simulink library "VIS_LIB"  (Simulink 8.6)
settings: Solver=ode45  StartTime=0.0  StopTime=10.0  RelTol=1e-3
undefined symbols (not defined in the file): AC, SIXOSEM_F_WD_AC_MASTER
libraries: cdsFilt x376, cdsEpicsOut x253, cdsEpicsIn x179, cdsTP x123, VIS_LIB x95, cdsMuxMatrix x91, cdsEpicsStringIn x75, cdsFiltCtrl x72, cdsFunctionCall x70, cdsRms x59, KAGRA_UTIL x25, STATE_BIO_MASTER x5
(part 30 of 38)

== system VIS_LIB/MODAL/inputproc_forQUA/OL_PROC ==
  MNSEG1 : Inport
  MNSEG2 : Inport  Port=2
  MNSEG3 : Inport  Port=3
  MNSEG4 : Inport  Port=4
  TILT_SEG1 : Inport  Port=5
  TILT_SEG2 : Inport  Port=6
  TILT_SEG3 : Inport  Port=7
  TILT_SEG4 : Inport  Port=8
  LEN_SEG1 : Inport  Port=9
  LEN_SEG2 : Inport  Port=10
  LEN_SEG3 : Inport  Port=11
  LEN_SEG4 : Inport  Port=12
  MN_TILT : VIS_LIB/UTILs/OL
  TM_LEN : VIS_LIB/UTILs/OL
  TM_TILT : VIS_LIB/UTILs/OL
  MNV : Outport
  MNH : Outport  Port=2
  TMV1 : Outport  Port=3
  TMV2 : Outport  Port=4
  TMH1 : Outport  Port=5
  TMH2 : Outport  Port=6
  wires:
  MNSEG2/1 -> MN_TILT/2
  MNSEG1/1 -> MN_TILT/1
  MNSEG4/1 -> MN_TILT/4
  MN_TILT/1 -> MNV/1
  MN_TILT/2 -> MNH/1
  MNSEG3/1 -> MN_TILT/3
  TILT_SEG1/1 -> TM_TILT/1
  TILT_SEG2/1 -> TM_TILT/2
  TILT_SEG4/1 -> TM_TILT/4
  TILT_SEG3/1 -> TM_TILT/3
  LEN_SEG1/1 -> TM_LEN/1
  LEN_SEG2/1 -> TM_LEN/2
  LEN_SEG3/1 -> TM_LEN/3
  LEN_SEG4/1 -> TM_LEN/4
  TM_TILT/1 -> TMV1/1
  TM_TILT/2 -> TMH1/1
  TM_LEN/1 -> TMV2/1
  TM_LEN/2 -> TMH2/1

== system VIS_LIB/MODAL/inputproc_forQUA/SEN2EUL ==
  In1 : Inport
  In2 : Inport  Port=2
  In3 : Inport  Port=3
  In4 : Inport  Port=4
  In5 : Inport  Port=5
  In6 : Inport  Port=6
  In7 : Inport  Port=7
  In8 : Inport  Port=8
  In9 : Inport  Port=9
  In10 : Inport  Port=10
  In11 : Inport  Port=11
  In12 : Inport  Port=12
  In13 : Inport  Port=13
  In14 : Inport  Port=14
  In15 : Inport  Port=15
  In20 : Inport  Port=16
  In21 : Inport  Port=17
  In22 : Inport  Port=18
  In27 : Inport  Port=19
  In28 : Inport  Port=20
  In29 : Inport  Port=21
  In30 : Inport  Port=22
  In31 : Inport  Port=23
  In32 : Inport  Port=24
  In33 : Inport  Port=25
  In34 : Inport  Port=26
  In35 : Inport  Port=27
  In36 : Inport  Port=28
  In37 : Inport  Port=29
  In38 : Inport  Port=30
  In16 : Inport  Port=31
  In17 : Inport  Port=32
  In18 : Inport  Port=33
  In19 : Inport  Port=34
  In23 : Inport  Port=35
  In24 : Inport  Port=36
  BF : cdsMuxMatrix/Subsystem  Tag=cdsMuxMatrix  Description=Any size matrix. Inputs and outputs must be connected using Mux and Demux parts.
      settings: AttributesFormatString=%<Tag>
  Demux{1..6} (6 alike) : Demux  Outputs=6
  IM : cdsMuxMatrix/Subsystem  Tag=cdsMuxMatrix  Description=Any size matrix. Inputs and outputs must be connected using Mux and Demux parts.
      settings: AttributesFormatString=%<Tag>
  IP : cdsMuxMatrix/Subsystem  Tag=cdsMuxMatrix  Description=Any size matrix. Inputs and outputs must be connected using Mux and Demux parts.
      settings: AttributesFormatString=%<Tag>
  MN : cdsMuxMatrix/Subsystem  Tag=cdsMuxMatrix  Description=Any size matrix. Inputs and outputs must be connected using Mux and Demux parts.
      settings: AttributesFormatString=%<Tag>
  MNOL : cdsMuxMatrix/Subsystem  Tag=cdsMuxMatrix  Description=Any size matrix. Inputs and outputs must be connected using Mux and Demux parts.
      settings: AttributesFormatString=%<Tag>
  Mux{1..6} (6 alike) : Mux  Inputs=6
  TM : cdsMuxMatrix/Subsystem  Tag=cdsMuxMatrix  Description=Any size matrix. Inputs and outputs must be connected using Mux and Demux parts.
      settings: AttributesFormatString=%<Tag>
  IPLo : Outport
  IPTo : Outport  Port=2
  IPVo : Outport  Port=3
  IPRo : Outport  Port=4
  IPPo : Outport  Port=5
  IPYo : Outport  Port=6
  BFLo : Outport  Port=7
  BFTo : Outport  Port=8
  BFVo : Outport  Port=9
  BFRo : Outport  Port=10
  BFPo : Outport  Port=11
  BFYo : Outport  Port=12
  MNLo : Outport  Port=13
  MNTo : Outport  Port=14
  MNVo : Outport  Port=15
  MNRo : Outport  Port=16
  MNPo : Outport  Port=17
  MNYo : Outport  Port=18
  IMLo : Outport  Port=19
  IMTo : Outport  Port=20
  IMVo : Outport  Port=21
  IMRo : Outport  Port=22
  IMPo : Outport  Port=23
  IMYo : Outport  Port=24
  TMLo : Outport  Port=25
  TMTo : Outport  Port=26
  TMVo : Outport  Port=27
  TMRo : Outport  Port=28
  TMPop : Outport  Port=29
  TMYo : Outport  Port=30
  TMLo1 : Outport  Port=31
  TMTo1 : Outport  Port=32
  TMVo1 : Outport  Port=33
  TMRo1 : Outport  Port=34
  TMPop1 : Outport  Port=35
  TMYo1 : Outport  Port=36
  wires:
  In6/1 -> Mux2/6
  Mux2/1 -> IP/1
  In3/1 -> Mux2/3
  In1/1 -> Mux2/1
  IP/1 -> Demux3/1
  In5/1 -> Mux2/5
  In2/1 -> Mux2/2
  In4/1 -> Mux2/4
  In12/1 -> Mux1/6
  Mux1/1 -> BF/1
  In9/1 -> Mux1/3
  In7/1 -> Mux1/1
  BF/1 -> Demux1/1
  In11/1 -> Mux1/5
  In8/1 -> Mux1/2
  In10/1 -> Mux1/4
  Mux3/1 -> MN/1
  In15/1 -> Mux3/3
  In13/1 -> Mux3/1
  MN/1 -> Demux2/1
  In14/1 -> Mux3/2
  Mux4/1 -> IM/1
  IM/1 -> Demux4/1
  In21/1 -> Mux3/5
  In20/1 -> Mux3/4
  In22/1 -> Mux3/6
  In30/1 -> Mux4/4
  In27/1 -> Mux4/1
  In29/1 -> Mux4/3
  In28/1 -> Mux4/2
  In32/1 -> Mux4/6
  In31/1 -> Mux4/5
  In38/1 -> Mux5/6
  Mux5/1 -> TM/1
  In35/1 -> Mux5/3
  In33/1 -> Mux5/1
  TM/1 -> Demux5/1
  In37/1 -> Mux5/5
  In34/1 -> Mux5/2
  In36/1 -> Mux5/4
  Demux3/6 -> IPYo/1
  Demux1/1 -> BFLo/1
  Demux1/2 -> BFTo/1
  Demux1/3 -> BFVo/1
  Demux1/4 -> BFRo/1
  Demux1/5 -> BFPo/1
  Demux1/6 -> BFYo/1
  Demux2/1 -> MNLo/1
  Demux2/2 -> MNTo/1
  Demux2/3 -> MNVo/1
  Demux2/4 -> MNRo/1
  Demux2/5 -> MNPo/1
  Demux2/6 -> MNYo/1
  Demux4/1 -> IMLo/1
  Demux4/2 -> IMTo/1
  Demux4/3 -> IMVo/1
  Demux4/4 -> IMRo/1
  Demux4/5 -> IMPo/1
  Demux4/6 -> IMYo/1
  Demux5/1 -> TMLo/1
  Demux3/1 -> IPLo/1
  Demux3/2 -> IPTo/1
  Demux3/3 -> IPVo/1
  Demux3/4 -> IPRo/1
  Demux3/5 -> IPPo/1
  Demux5/2 -> TMTo/1
  Demux5/3 -> TMVo/1
  Demux5/4 -> TMRo/1
  Demux5/5 -> TMPop/1
  Demux5/6 -> TMYo/1
  In24/1 -> Mux6/6
  Mux6/1 -> MNOL/1
  In18/1 -> Mux6/3
  MNOL/1 -> Demux6/1
  In23/1 -> Mux6/5
  In17/1 -> Mux6/2
  In19/1 -> Mux6/4
  Demux6/2 -> TMTo1/1
  Demux6/3 -> TMVo1/1
  Demux6/4 -> TMRo1/1
  Demux6/5 -> TMPop1/1
  Demux6/6 -> TMYo1/1
  Demux6/1 -> TMLo1/1
  In16/1 -> Mux6/1

== system VIS_LIB/MODAL/inputproc_forQUA/SENSIN ==
  IPLVDT_H1 : Inport
  IPLVDT_H2 : Inport  Port=2
  IPLVDT_H3 : Inport  Port=3
  BFLVDT_V1 : Inport  Port=4
  BFLVDT_V2 : Inport  Port=5
  BFLVDT_V3 : Inport  Port=6
  BFLVDT_H1 : Inport  Port=7
  BFLVDT_H2 : Inport  Port=8
  BFLVDT_H3 : Inport  Port=9
  MCPS_V1 : Inport  Port=10
  MCPS_V2 : Inport  Port=11
  MCPS_V3 : Inport  Port=12
  MCPS_H1 : Inport  Port=13
  MCPS_H2 : Inport  Port=14
  MNPS_H3 : Inport  Port=15
  IMPS_V1 : Inport  Port=16
  IMPS_V2 : Inport  Port=17
  IMPS_V3 : Inport  Port=18
  IMPS_H1 : Inport  Port=19
  IMPS_H2 : Inport  Port=20
  IMPS_H3 : Inport  Port=21
  MNOL_V : Inport  Port=22
  MNOL_H4 : Inport  Port=23
  TMOLV1 : Inport  Port=24
  TMOLV2 : Inport  Port=25
  TMOLH1 : Inport  Port=26
  TMOLH2 : Inport  Port=27
  BF : VIS_LIB/UTILs/6COILs_DQ
  Ground{1..7,9..10} (9 alike) : Ground
  IM : VIS_LIB/UTILs/6COILs_DQ
  IP : VIS_LIB/UTILs/6COILs_DQ
  MN : VIS_LIB/UTILs/6COILs_DQ
  MNOL : VIS_LIB/UTILs/6COILs_DQ
  TM : VIS_LIB/UTILs/6COILs_DQ
  IPV1 : Outport
  IPV2 : Outport  Port=2
  IPV3 : Outport  Port=3
  IPH1 : Outport  Port=4
  IPH2 : Outport  Port=5
  IPH3 : Outport  Port=6
  BFV1 : Outport  Port=7
  BFV2 : Outport  Port=8
  BFV3 : Outport  Port=9
  BFH1 : Outport  Port=10
  BFH2 : Outport  Port=11
  BFH3 : Outport  Port=12
  MNV1 : Outport  Port=13
  MNV2 : Outport  Port=14
  MNV3 : Outport  Port=15
  MNH1 : Outport  Port=16
  MNH2 : Outport  Port=17
  MNH3 : Outport  Port=18
  IMV1 : Outport  Port=19
  IMV2 : Outport  Port=20
  IMV3 : Outport  Port=21
  IMH1 : Outport  Port=22
  IMH2 : Outport  Port=23
  IMH3 : Outport  Port=24
  IMV4 : Outport  Port=25
  IMV5 : Outport  Port=26
  IMV6 : Outport  Port=27
  IMH4 : Outport  Port=28
  IMH5 : Outport  Port=29
  IMH6 : Outport  Port=30
  MNOLV1 : Outport  Port=31
  MNOLV2 : Outport  Port=32
  MNOLV3 : Outport  Port=33
  MNOLH1 : Outport  Port=34
  MNOLH2 : Outport  Port=35
  MNOLH3 : Outport  Port=36
  wires:
  IPLVDT_H1/1 -> IP/4
  IPLVDT_H2/1 -> IP/5
  IPLVDT_H3/1 -> IP/6
  BFLVDT_V1/1 -> BF/1
  BFLVDT_V2/1 -> BF/2
  BFLVDT_V3/1 -> BF/3
  BFLVDT_H1/1 -> BF/4
  BFLVDT_H2/1 -> BF/5
  BFLVDT_H3/1 -> BF/6
  MCPS_V1/1 -> MN/1
  MCPS_V2/1 -> MN/2
  MCPS_V3/1 -> MN/3
  MCPS_H1/1 -> MN/4
  MCPS_H2/1 -> MN/5
  MNPS_H3/1 -> MN/6
  IMPS_V1/1 -> IM/1
  IMPS_V2/1 -> IM/2
  IMPS_V3/1 -> IM/3
  IMPS_H1/1 -> IM/4
  IMPS_H2/1 -> IM/5
  IMPS_H3/1 -> IM/6
  Ground2/1 -> IP/1
  Ground1/1 -> IP/2
  Ground3/1 -> IP/3
  IP/5 -> IPH2/1
  IP/4 -> IPH1/1
  IP/6 -> IPH3/1
  BF/1 -> BFV1/1
  BF/3 -> BFV3/1
  BF/5 -> BFH2/1
  BF/6 -> BFH3/1
  BF/2 -> BFV2/1
  BF/4 -> BFH1/1
  IM/6 -> IMH3/1
  IM/5 -> IMH2/1
  IM/4 -> IMH1/1
  IM/3 -> IMV3/1
  IM/2 -> IMV2/1
  IM/1 -> IMV1/1
  MN/6 -> MNH3/1
  MN/5 -> MNH2/1
  MN/4 -> MNH1/1
  MN/3 -> MNV3/1
  MN/2 -> MNV2/1
  MN/1 -> MNV1/1
  IP/1 -> IPV1/1
  IP/2 -> IPV2/1
  IP/3 -> IPV3/1
  MNOL_V/1 -> MNOL/1
  MNOL_H4/1 -> MNOL/4
  TMOLV2/1 -> TM/2
  TMOLH1/1 -> TM/4
  TMOLH2/1 -> TM/5
  TM/6 -> IMH6/1
  TM/5 -> IMH5/1
  TM/4 -> IMH4/1
  TM/3 -> IMV6/1
  TM/2 -> IMV5/1
  TMOLV1/1 -> TM/1
  Ground9/1 -> TM/3
  Ground10/1 -> TM/6
  TM/1 -> IMV4/1
  MNOL/6 -> MNOLH3/1
  MNOL/5 -> MNOLH2/1
  MNOL/4 -> MNOLH1/1
  MNOL/3 -> MNOLV3/1
  MNOL/2 -> MNOLV2/1
  Ground5/1 -> MNOL/3
  Ground4/1 -> MNOL/6
  MNOL/1 -> MNOLV1/1
  Ground7/1 -> MNOL/2
  Ground6/1 -> MNOL/5

== system VIS_LIB/MODAL/inputproc_forQUA/SENSIN_GAS ==
  note: #DAQ Channels
      |
      | F0_OUT 256
      | F1_OUT 256
      | F2_OUT 256
      | F3_OUT 256
      | BF_OUT 256
  iF0 : Inport
  iF1 : Inport  Port=2
  iF2 : Inport  Port=3
  iF3 : Inport  Port=4
  iBF : Inport  Port=5
  BF : cdsFilt/Subsystem  Tag=cdsFilt  Description=|
      | Purpose:                                                                                                                                                                                                                                  
      | Standard CDS IIR filter module.                                                                                                                                                                                                           
      |                                                                                                                                                                                                                                           
      | Operation:                                                                                                                                                                                                                                
      | Consists of 10 second order section IIR filters, plus a ramped gain stage. In FE code, also provides pre-defined test points and excitation channel inputs. The filter coefficients are defined in the LIGO system using the 'foton' tool.
      |                                                                                                                                                                                                                                           
      | Usage:                                                                                                                                                                                                                                    
      | Name the part with the desired filter module name.
      settings: AttributesFormatString=%<Tag>
  F0 : cdsFilt/Subsystem  Tag=cdsFilt  Description=|
      | Purpose:                                                                                                                                                                                                                                  
      | Standard CDS IIR filter module.                                                                                                                                                                                                           
      |                                                                                                                                                                                                                                           
      | Operation:                                                                                                                                                                                                                                
      | Consists of 10 second order section IIR filters, plus a ramped gain stage. In FE code, also provides pre-defined test points and excitation channel inputs. The filter coefficients are defined in the LIGO system using the 'foton' tool.
      |                                                                                                                                                                                                                                           
      | Usage:                                                                                                                                                                                                                                    
      | Name the part with the desired filter module name.
      settings: AttributesFormatString=%<Tag>
  F1 : cdsFilt/Subsystem  Tag=cdsFilt  Description=|
      | Purpose:                                                                                                                                                                                                                                  
      | Standard CDS IIR filter module.                                                                                                                                                                                                           
      |                                                                                                                                                                                                                                           
      | Operation:                                                                                                                                                                                                                                
      | Consists of 10 second order section IIR filters, plus a ramped gain stage. In FE code, also provides pre-defined test points and excitation channel inputs. The filter coefficients are defined in the LIGO system using the 'foton' tool.
      |                                                                                                                                                                                                                                           
      | Usage:                                                                                                                                                                                                                                    
      | Name the part with the desired filter module name.
      settings: AttributesFormatString=%<Tag>
  F2 : cdsFilt/Subsystem  Tag=cdsFilt  Description=|
      | Purpose:                                                                                                                                                                                                                                  
      | Standard CDS IIR filter module.                                                                                                                                                                                                           
      |                                                                                                                                                                                                                                           
      | Operation:                                                                                                                                                                                                                                
      | Consists of 10 second order section IIR filters, plus a ramped gain stage. In FE code, also provides pre-defined test points and excitation channel inputs. The filter coefficients are defined in the LIGO system using the 'foton' tool.
      |                                                                                                                                                                                                                                           
      | Usage:                                                                                                                                                                                                                                    
      | Name the part with the desired filter module name.
      settings: AttributesFormatString=%<Tag>
  F3 : cdsFilt/Subsystem  Tag=cdsFilt  Description=|
      | Purpose:                                                                                                                                                                                                                                  
      | Standard CDS IIR filter module.                                                                                                                                                                                                           
      |                                                                                                                                                                                                                                           
      | Operation:                                                                                                                                                                                                                                
      | Consists of 10 second order section IIR filters, plus a ramped gain stage. In FE code, also provides pre-defined test points and excitation channel inputs. The filter coefficients are defined in the LIGO system using the 'foton' tool.
      |                                                                                                                                                                                                                                           
      | Usage:                                                                                                                                                                                                                                    
      | Name the part with the desired filter module name.
      settings: AttributesFormatString=%<Tag>
  oF0 : Outport
  oF1 : Outport  Port=2
  oF2 : Outport  Port=3
  oF3 : Outport  Port=4
  oBF : Outport  Port=5
  wires:
  BF/1 -> oBF/1
  iBF/1 -> BF/1
  F3/1 -> oF3/1
  iF3/1 -> F3/1
  F2/1 -> oF2/1
  iF2/1 -> F2/1
  F1/1 -> oF1/1
  iF1/1 -> F1/1
  F0/1 -> oF0/1
  iF0/1 -> F0/1

== system VIS_LIB/WD2/AC/BANDLIM ==
  F0_In : Inport
  SF_In : Inport  Port=2
  BF_In : Inport  Port=3
  BF : cdsFilt/Subsystem  Tag=cdsFilt  Description=|
      | Purpose:                                                                                                                                                                                                                                  
      | Standard CDS IIR filter module.                                                                                                                                                                                                           
      |                                                                                                                                                                                                                                           
      | Operation:                                                                                                                                                                                                                                
      | Consists of 10 second order section IIR filters, plus a ramped gain stage. In FE code, also provides pre-defined test points and excitation channel inputs. The filter coefficients are defined in the LIGO system using the 'foton' tool.
      |                                                                                                                                                                                                                                           
      | Usage:                                                                                                                                                                                                                                    
      | Name the part with the desired filter module name.
      settings: AttributesFormatString=%<Tag>
  F0 : cdsFilt/Subsystem  Tag=cdsFilt  Description=|
      | Purpose:                                                                                                                                                                                                                                  
      | Standard CDS IIR filter module.                                                                                                                                                                                                           
      |                                                                                                                                                                                                                                           
      | Operation:                                                                                                                                                                                                                                
      | Consists of 10 second order section IIR filters, plus a ramped gain stage. In FE code, also provides pre-defined test points and excitation channel inputs. The filter coefficients are defined in the LIGO system using the 'foton' tool.
      |                                                                                                                                                                                                                                           
      | Usage:                                                                                                                                                                                                                                    
      | Name the part with the desired filter module name.
      settings: AttributesFormatString=%<Tag>
  SF : cdsFilt/Subsystem  Tag=cdsFilt  Description=|
      | Purpose:                                                                                                                                                                                                                                  
      | Standard CDS IIR filter module.                                                                                                                                                                                                           
      |                                                                                                                                                                                                                                           
      | Operation:                                                                                                                                                                                                                                
      | Consists of 10 second order section IIR filters, plus a ramped gain stage. In FE code, also provides pre-defined test points and excitation channel inputs. The filter coefficients are defined in the LIGO system using the 'foton' tool.
      |                                                                                                                                                                                                                                           
      | Usage:                                                                                                                                                                                                                                    
      | Name the part with the desired filter module name.
      settings: AttributesFormatString=%<Tag>
  F0_Out : Outport
  SF_Out : Outport  Port=2
  BF_Out : Outport  Port=3
  wires:
  BF/1 -> BF_Out/1
  BF_In/1 -> BF/1
  SF/1 -> SF_Out/1
  SF_In/1 -> SF/1
  F0/1 -> F0_Out/1
  F0_In/1 -> F0/1

== system VIS_LIB/WD3/OSEMAC/BANDLIM ==
  V1_In : Inport
  V2_In : Inport  Port=2
  V3_In : Inport  Port=3
  H1_In : Inport  Port=4
  H2_In : Inport  Port=5
  H3_In : Inport  Port=6
  H1 : cdsFilt/Subsystem  Tag=cdsFilt  Description=|
      | Purpose:                                                                                                                                                                                                                                  
      | Standard CDS IIR filter module.                                                                                                                                                                                                           
      |                                                                                                                                                                                                                                           
      | Operation:                                                                                                                                                                                                                                
      | Consists of 10 second order section IIR filters, plus a ramped gain stage. In FE code, also provides pre-defined test points and excitation channel inputs. The filter coefficients are defined in the LIGO system using the 'foton' tool.
      |                                                                                                                                                                                                                                           
      | Usage:                                                                                                                                                                                                                                    
      | Name the part with the desired filter module name.
      settings: AttributesFormatString=%<Tag>
  H2 : cdsFilt/Subsystem  Tag=cdsFilt  Description=|
      | Purpose:                                                                                                                                                                                                                                  
      | Standard CDS IIR filter module.                                                                                                                                                                                                           
      |                                                                                                                                                                                                                                           
      | Operation:                                                                                                                                                                                                                                
      | Consists of 10 second order section IIR filters, plus a ramped gain stage. In FE code, also provides pre-defined test points and excitation channel inputs. The filter coefficients are defined in the LIGO system using the 'foton' tool.
      |                                                                                                                                                                                                                                           
      | Usage:                                                                                                                                                                                                                                    
      | Name the part with the desired filter module name.
      settings: AttributesFormatString=%<Tag>
  H3 : cdsFilt/Subsystem  Tag=cdsFilt  Description=|
      | Purpose:                                                                                                                                                                                                                                  
      | Standard CDS IIR filter module.                                                                                                                                                                                                           
      |                                                                                                                                                                                                                                           
      | Operation:                                                                                                                                                                                                                                
      | Consists of 10 second order section IIR filters, plus a ramped gain stage. In FE code, also provides pre-defined test points and excitation channel inputs. The filter coefficients are defined in the LIGO system using the 'foton' tool.
      |                                                                                                                                                                                                                                           
      | Usage:                                                                                                                                                                                                                                    
      | Name the part with the desired filter module name.
      settings: AttributesFormatString=%<Tag>
  V1 : cdsFilt/Subsystem  Tag=cdsFilt  Description=|
      | Purpose:                                                                                                                                                                                                                                  
      | Standard CDS IIR filter module.                                                                                                                                                                                                           
      |                                                                                                                                                                                                                                           
      | Operation:                                                                                                                                                                                                                                
      | Consists of 10 second order section IIR filters, plus a ramped gain stage. In FE code, also provides pre-defined test points and excitation channel inputs. The filter coefficients are defined in the LIGO system using the 'foton' tool.
      |                                                                                                                                                                                                                                           
      | Usage:                                                                                                                                                                                                                                    
      | Name the part with the desired filter module name.
      settings: AttributesFormatString=%<Tag>
  V2 : cdsFilt/Subsystem  Tag=cdsFilt  Description=|
      | Purpose:                                                                                                                                                                                                                                  
      | Standard CDS IIR filter module.                                                                                                                                                                                                           
      |                                                                                                                                                                                                                                           
      | Operation:                                                                                                                                                                                                                                
      | Consists of 10 second order section IIR filters, plus a ramped gain stage. In FE code, also provides pre-defined test points and excitation channel inputs. The filter coefficients are defined in the LIGO system using the 'foton' tool.
      |                                                                                                                                                                                                                                           
      | Usage:                                                                                                                                                                                                                                    
      | Name the part with the desired filter module name.
      settings: AttributesFormatString=%<Tag>
  V3 : cdsFilt/Subsystem  Tag=cdsFilt  Description=|
      | Purpose:                                                                                                                                                                                                                                  
      | Standard CDS IIR filter module.                                                                                                                                                                                                           
      |                                                                                                                                                                                                                                           
      | Operation:                                                                                                                                                                                                                                
      | Consists of 10 second order section IIR filters, plus a ramped gain stage. In FE code, also provides pre-defined test points and excitation channel inputs. The filter coefficients are defined in the LIGO system using the 'foton' tool.
      |                                                                                                                                                                                                                                           
      | Usage:                                                                                                                                                                                                                                    
      | Name the part with the desired filter module name.
      settings: AttributesFormatString=%<Tag>
  V1_Out : Outport
  V2_Out : Outport  Port=2
  V3_Out : Outport  Port=3
  H1_Out : Outport  Port=4
  H2_Out : Outport  Port=5
  H3_Out : Outport  Port=6
  wires:
  V1/1 -> V1_Out/1
  V2/1 -> V2_Out/1
  V3/1 -> V3_Out/1
  V1_In/1 -> V1/1
  V2_In/1 -> V2/1
  V3_In/1 -> V3/1
  H1/1 -> H1_Out/1
  H2/1 -> H2_Out/1
  H3/1 -> H3_Out/1
  H1_In/1 -> H1/1
  H2_In/1 -> H2/1
  H3_In/1 -> H3/1

== system VIS_LIB/WD4/AC/BANDLIM ==
  SF_In : Inport
  BF_In : Inport  Port=2
  BF : cdsFilt/Subsystem  Tag=cdsFilt  Description=|
      | Purpose:                                                                                                                                                                                                                                  
      | Standard CDS IIR filter module.                                                                                                                                                                                                           
      |                                                                                                                                                                                                                                           
      | Operation:                                                                                                                                                                                                                                
      | Consists of 10 second order section IIR filters, plus a ramped gain stage. In FE code, also provides pre-defined test points and excitation channel inputs. The filter coefficients are defined in the LIGO system using the 'foton' tool.
      |                                                                                                                                                                                                                                           
      | Usage:                                                                                                                                                                                                                                    
      | Name the part with the desired filter module name.
      settings: AttributesFormatString=%<Tag>
  SF : cdsFilt/Subsystem  Tag=cdsFilt  Description=|
      | Purpose:                                                                                                                                                                                                                                  
      | Standard CDS IIR filter module.                                                                                                                                                                                                           
      |                                                                                                                                                                                                                                           
      | Operation:                                                                                                                                                                                                                                
      | Consists of 10 second order section IIR filters, plus a ramped gain stage. In FE code, also provides pre-defined test points and excitation channel inputs. The filter coefficients are defined in the LIGO system using the 'foton' tool.
      |                                                                                                                                                                                                                                           
      | Usage:                                                                                                                                                                                                                                    
      | Name the part with the desired filter module name.
      settings: AttributesFormatString=%<Tag>
  SF_Out : Outport
  BF_Out : Outport  Port=2
  wires:
  BF/1 -> BF_Out/1
  BF_In/1 -> BF/1
  SF/1 -> SF_Out/1
  SF_In/1 -> SF/1
